simulink library "tetherDragForceNEqual2_ul"  (R2018b)
settings: Solver=VariableStepAuto  StartTime=0.0  StopTime=10.0  RelTol=1e-3
values from neighbouring files (symbols this model uses):
  Cd = 0.5    [tetherDragForce_ts.m]
  dia_t = 0.01    [tetherDragForce_ts.m]
  N = 5    [tetherDragForce_ts.m]
  rho_fluid = 1000    [tetherDragForce_ts.m]
settings Model: Creator=asiddiq2  LastModifiedBy=Ayaz

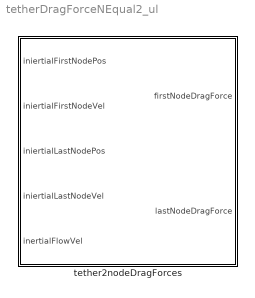
== system tetherDragForceNEqual2_ul ==
  tether2nodeDragForces : Subsystem  mask{dia_t=dia_t, Cd=Cd, rho_fluid=rho_fluid}
      mask prompts: dia_t "Tether diameter"; Cd "Tether drag coefficient"; rho_fluid "Fluid density (kg/m^3)"

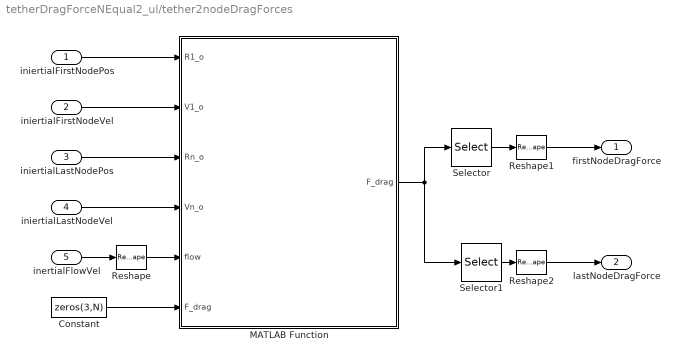
== system tetherDragForceNEqual2_ul/tether2nodeDragForces ==
  iniertialFirstNodePos : Inport
  iniertialFirstNodeVel : Inport  Port=2
  iniertialLastNodePos : Inport  Port=3
  iniertialLastNodeVel : Inport  Port=4
  inertialFlowVel : Inport  Port=5
  Constant : Constant  Value=zeros(3,N)
  MATLAB Function : MATLAB Function  TreatAsAtomicUnit=on
  Reshape : Reshape  OutputDimensionality=Column vector (2-D)
  Reshape1 : Reshape  OutputDimensionality=Column vector (2-D)
  Reshape2 : Reshape  OutputDimensionality=Column vector (2-D)
  Selector : Selector  NumberOfDimensions=2  InputPortWidth=3  IndexOptions=Select all,Index vector (dialog)  Indices=[1 3],1  OutputSizes=1,1
  Selector1 : Selector  NumberOfDimensions=2  InputPortWidth=3  IndexOptions=Select all,Index vector (dialog)  Indices=[1 3],N  OutputSizes=1,1
  firstNodeDragForce : Outport
  lastNodeDragForce : Outport  Port=2
  wires:
  inertialFlowVel/1 -> Reshape/1
  Constant/1 -> MATLAB Function/6("F_drag ")
  Reshape/1 -> MATLAB Function/5(flow)
  iniertialLastNodeVel/1 -> MATLAB Function/4(Vn_o)
  iniertialLastNodePos/1 -> MATLAB Function/3(Rn_o)
  iniertialFirstNodeVel/1 -> MATLAB Function/2(V1_o)
  iniertialFirstNodePos/1 -> MATLAB Function/1(R1_o)
  MATLAB Function/1(F_drag) -> Selector1/1, Selector/1
  Selector/1 -> Reshape1/1
  Reshape1/1 -> firstNodeDragForce/1
  Selector1/1 -> Reshape2/1
  Reshape2/1 -> lastNodeDragForce/1

== matlab function tetherDragForceNEqual2_ul/tether2nodeDragForces/MATLAB Function ==
  data: R1_o input; V1_o input; Rn_o input; Vn_o input; F_drag output; flow input; F_drag input; Cd parameter; rho_fluid parameter; N parameter; dia_t parameter
function F_drag = fcn(R1_o,V1_o,Rn_o,Vn_o,flow,F_drag,Cd, rho_fluid,N, dia_t)

Ri_o = [R1_o Rn_o];
Vi_o = [V1_o Vn_o];

Ve = zeros(3,N-1);
Vrel = zeros(3,N-1);
drag_direction = zeros(3,N-1);
drag = zeros(3,N-1);

qe = zeros(N-1,1);
di = zeros(N-1,1);
th = zeros(N-1,1);
S = zeros(N-1,1);

% elemental velocity
for i = 1:N-1
    
    % relative velocity
    Ve(:,i) = (Vi_o(:,i) + Vi_o(:,i+1))/2;
    Vrel(:,i) = flow - Ve(:,i);
    Vrel(3,i) = 0;
    % drag direction
    if norm(Vrel(:,i)) > 1e-3
        drag_direction(:,i) = Vrel(:,i)/norm(Vrel(:,i));
    else
        drag_direction(:,i) = zeros(3,1);
    end
    
    % dynamic pressure
    qe(i) = 0.5*rho_fluid*norm(Vrel(:,i))^2;
    
    % projected area
    di(i) = norm(Ri_o(:,i+1)-Ri_o(:,i));
    th(i) = atan( (Ri_o(3,i+1)-Ri_o(3,i))/norm(Ri_o(1:2,i+1)-Ri_o(1:2,i)) );
    S(i) = di(i)*dia_t*sin(th(i));
    
    drag(:,i) = 0.5*rho_fluid*Cd*Vrel(:,i)*norm(Vrel(:,i))*S(i);
end

% drag force acting on each node'
for i = 1:N
    if i == 1
        F_drag(:,i) = drag(:,i)/2;
    elseif i == N
        F_drag(:,i) = drag(:,i-1)/2;
    end
end

end
